simulink model "athree_phase_transestor_converter_hystersis"  (R2015a)
settings: Solver=ode45  StartTime=0.0  StopTime=0.1  RelTol=1e-3
libraries: simulink_extras x1
settings Model: Creator=Windows 10  LastModifiedBy=Windows 10

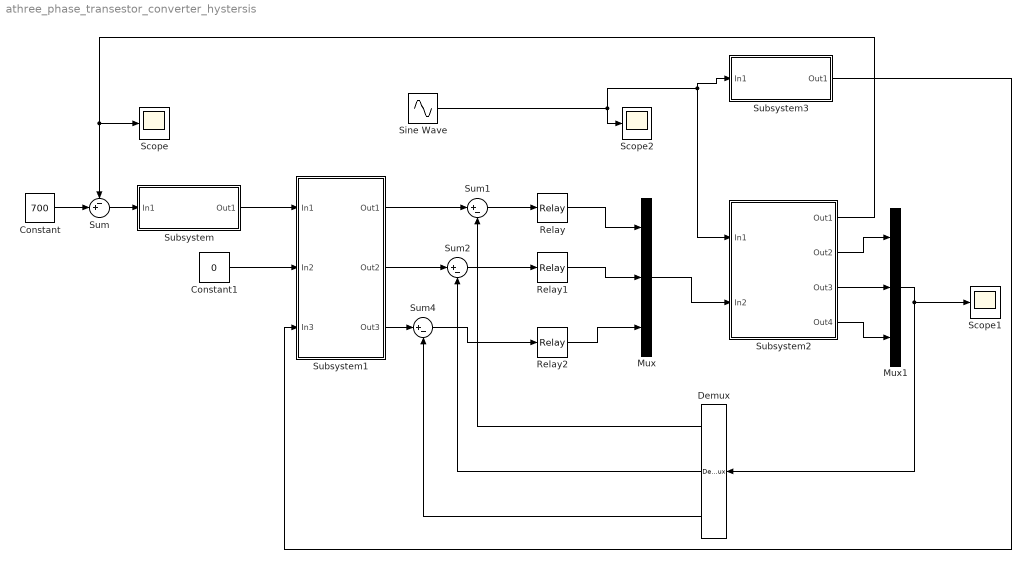
== system athree_phase_transestor_converter_hystersis ==
  Constant : Constant  Value=700
  Constant1 : Constant  Value=0
  Demux : Demux  Outputs=3
  Mux : Mux  Inputs=3
  Mux1 : Mux  Inputs=3
  Relay : Relay  OnSwitchValue=1  OffSwitchValue=-1  OnOutputValue=0  OffOutputValue=1
  Relay1 : Relay  OnSwitchValue=1  OffSwitchValue=-1  OnOutputValue=0  OffOutputValue=1
  Relay2 : Relay  OnSwitchValue=1  OffSwitchValue=-1  OnOutputValue=0  OffOutputValue=1
  Scope : Scope
  Scope1 : Scope
  Scope2 : Scope
      settings: SaveName=ScopeData2
  Sine Wave : Sin  Amplitude=326.5  Frequency=100*pi  Phase=[0 2*pi/3 4*pi/3]  SampleTime=0
  Subsystem : Subsystem
  Subsystem1 : Subsystem
  Subsystem2 : Subsystem
  Subsystem3 : Subsystem
  Sum : Sum  Inputs=-+|
  Sum1 : Sum  Inputs=|+-
  Sum2 : Sum  Inputs=|+-
  Sum4 : Sum  Inputs=|+-
  wires:
  Constant/1 -> Sum/2
  Sum/1 -> Subsystem/1(In1)
  Subsystem/1(Out1) -> Subsystem1/1(In1)
  Constant1/1 -> Subsystem1/2(In2)
  Subsystem1/1(Out1) -> Sum1/1
  Subsystem1/3(Out3) -> Sum4/1
  Subsystem1/2(Out2) -> Sum2/1
  Sum1/1 -> Relay/1
  Sum4/1 -> Relay2/1
  Sum2/1 -> Relay1/1
  Relay1/1 -> Mux/2
  Relay2/1 -> Mux/3
  Relay/1 -> Mux/1
  Demux/1 -> Sum1/2
  Demux/2 -> Sum2/2
  Demux/3 -> Sum4/2
  Subsystem3/1(Out1) -> Subsystem1/3(In3)
  Sine Wave/1 -> Subsystem3/1(In1), Subsystem2/1(In1), Scope2/1
  Mux/1 -> Subsystem2/2(In2)
  Subsystem2/2(Out2) -> Mux1/1
  Subsystem2/3(Out3) -> Mux1/2
  Subsystem2/4(Out4) -> Mux1/3
  Subsystem2/1(Out1) -> Sum/1, Scope/1
  Mux1/1 -> Scope1/1, Demux/1

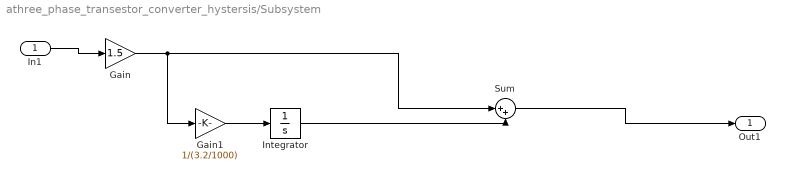
== system athree_phase_transestor_converter_hystersis/Subsystem ==
  In1 : Inport
  Gain : Gain  Gain=1.5
  Gain1 : Gain  Gain=1/(3.2/1000)
  Integrator : Integrator
  Sum : Sum  Inputs=|++
  Out1 : Outport
  wires:
  Gain1/1 -> Integrator/1
  Integrator/1 -> Sum/2
  Gain/1 -> Gain1/1, Sum/1
  In1/1 -> Gain/1
  Sum/1 -> Out1/1

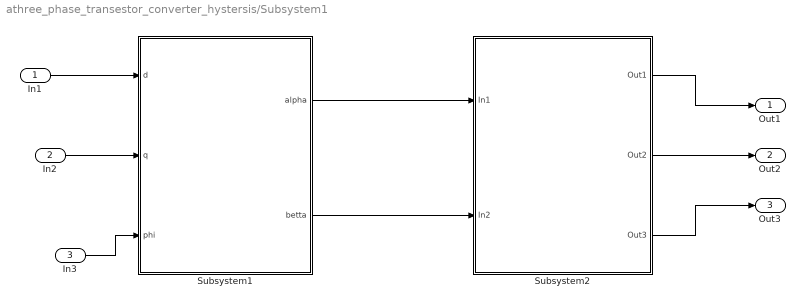
== system athree_phase_transestor_converter_hystersis/Subsystem1 ==
  In1 : Inport
  In2 : Inport  Port=2
  In3 : Inport  Port=3
  Subsystem1 : Subsystem
  Subsystem2 : Subsystem
  Out1 : Outport
  Out2 : Outport  Port=2
  Out3 : Outport  Port=3
  wires:
  Subsystem2/2(Out2) -> Out2/1
  Subsystem1/1(alpha) -> Subsystem2/1(In1)
  Subsystem2/3(Out3) -> Out3/1
  Subsystem2/1(Out1) -> Out1/1
  In3/1 -> Subsystem1/3(phi)
  In1/1 -> Subsystem1/1(d)
  In2/1 -> Subsystem1/2(q)
  Subsystem1/2(betta) -> Subsystem2/2(In2)

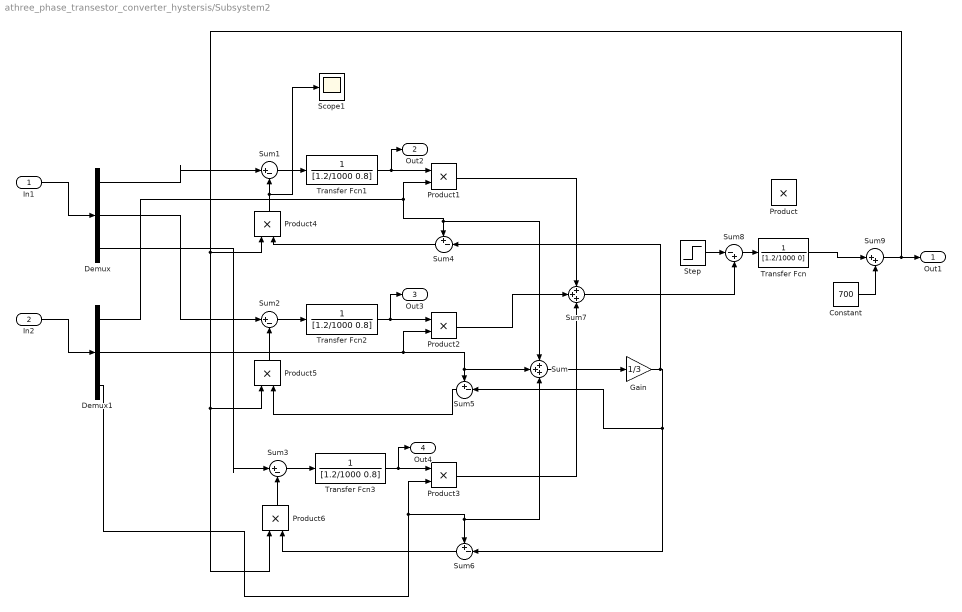
== system athree_phase_transestor_converter_hystersis/Subsystem2 ==
  In1 : Inport
  In2 : Inport  Port=2
  Constant : Constant  Value=700
  Demux : Demux  Outputs=3
  Demux1 : Demux  Outputs=3
  Gain : Gain  Gain=1/3
  Product{,1..6} (7 alike) : Product
  Scope1 : Scope
      settings: SaveName=ScopeData3
  Step : Step  Time=0.05  Before=15  After=30  SampleTime=0
  Sum : Sum  Inputs=+++
  Sum1 : Sum  Inputs=|+-
  Sum2 : Sum  Inputs=|+-
  Sum3 : Sum  Inputs=|+-
  Sum4 : Sum  Inputs=+-|
  Sum5 : Sum  Inputs=+-|
  Sum6 : Sum  Inputs=+-|
  Sum7 : Sum  Inputs=+++
  Sum8 : Sum  Inputs=|-+
  Sum9 : Sum  Inputs=|++
  Transfer Fcn : TransferFcn  Denominator=[1.2/1000 0]
  Transfer Fcn1 : TransferFcn  Denominator=[1.2/1000 0.8]
  Transfer Fcn2 : TransferFcn  Denominator=[1.2/1000 0.8]
  Transfer Fcn3 : TransferFcn  Denominator=[1.2/1000 0.8]
  Out1 : Outport
  Out2 : Outport  Port=2
  Out3 : Outport  Port=3
  Out4 : Outport  Port=4
  wires:
  In1/1 -> Demux/1
  In2/1 -> Demux1/1
  Sum1/1 -> Transfer Fcn1/1
  Sum2/1 -> Transfer Fcn2/1
  Sum3/1 -> Transfer Fcn3/1
  Demux/1 -> Sum1/1
  Demux/2 -> Sum2/1
  Demux/3 -> Sum3/1
  Transfer Fcn1/1 -> Out2/1, Product1/1
  Transfer Fcn2/1 -> Out3/1, Product2/1
  Transfer Fcn3/1 -> Out4/1, Product3/1
  Product4/1 -> Scope1/1, Sum1/2
  Product5/1 -> Sum2/2
  Product6/1 -> Sum3/2
  Demux1/1 -> Sum/1, Sum4/1, Product1/2
  Sum4/1 -> Product4/2
  Sum5/1 -> Product5/2
  Sum6/1 -> Product6/2
  Demux1/2 -> Sum/2, Sum5/1, Product2/2
  Demux1/3 -> Sum/3, Sum6/1, Product3/2
  Product2/1 -> Sum7/2
  Product1/1 -> Sum7/1
  Product3/1 -> Sum7/3
  Sum7/1 -> Sum8/2
  Step/1 -> Sum8/1
  Sum8/1 -> Transfer Fcn/1
  Transfer Fcn/1 -> Sum9/1
  Constant/1 -> Sum9/2
  Sum9/1 -> Product4/1, Product5/1, Product6/1, Out1/1
  Sum/1 -> Gain/1
  Gain/1 -> Sum4/2, Sum5/2, Sum6/2

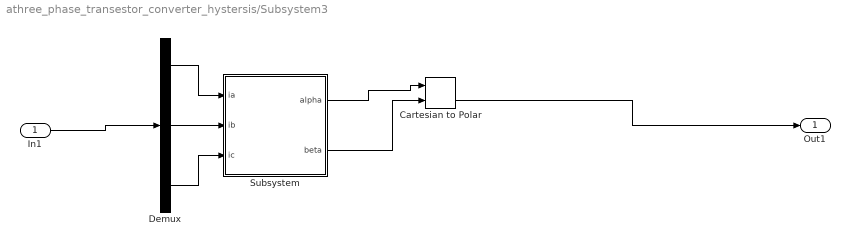
== system athree_phase_transestor_converter_hystersis/Subsystem3 ==
  In1 : Inport
  Cartesian to Polar : simulink_extras/Transformations/Cartesian to Polar
  Demux : Demux  Outputs=3
  Subsystem : Subsystem
  Out1 : Outport
  wires:
  Subsystem/1(alpha) -> Cartesian to Polar/1
  Subsystem/2(beta) -> Cartesian to Polar/2
  Cartesian to Polar/2 -> Out1/1
  In1/1 -> Demux/1
  Demux/1 -> Subsystem/1(ia)
  Demux/2 -> Subsystem/2(ib)
  Demux/3 -> Subsystem/3(ic)

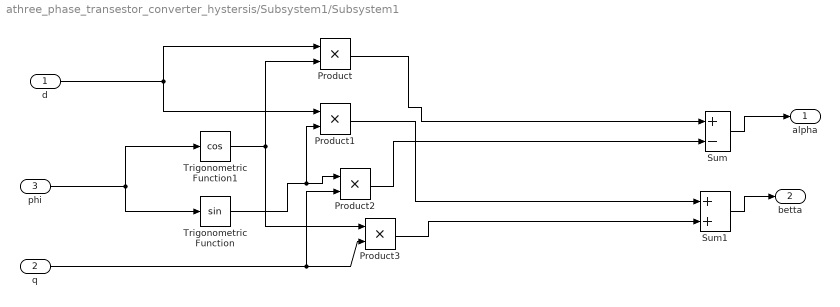
== system athree_phase_transestor_converter_hystersis/Subsystem1/Subsystem1 ==
  d : Inport
  q : Inport  Port=2
  phi : Inport  Port=3
  Product{,1..3} (4 alike) : Product
  Sum : Sum  Inputs=+-
  Sum1 : Sum
  Trigonometric Function : Trigonometry
  Trigonometric Function1 : Trigonometry  Operator=cos
  alpha : Outport
  betta : Outport  Port=2
  wires:
  Sum/1 -> alpha/1
  Sum1/1 -> betta/1
  phi/1 -> Trigonometric Function/1, Trigonometric Function1/1
  Product/1 -> Sum/1
  Product1/1 -> Sum1/1
  Product2/1 -> Sum/2
  Product3/1 -> Sum1/2
  q/1 -> Product2/2, Product3/2
  Trigonometric Function/1 -> Product1/2, Product2/1
  Trigonometric Function1/1 -> Product3/1, Product/2
  d/1 -> Product1/1, Product/1

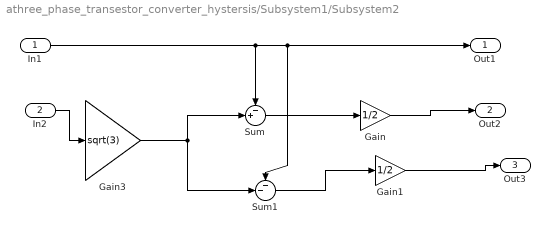
== system athree_phase_transestor_converter_hystersis/Subsystem1/Subsystem2 ==
  In1 : Inport
  In2 : Inport  Port=2
  Gain : Gain  Gain=1/2
  Gain1 : Gain  Gain=1/2
  Gain3 : Gain  Gain=sqrt(3)
  Sum : Sum  Inputs=-+|
  Sum1 : Sum  Inputs=--|
  Out1 : Outport
  Out2 : Outport  Port=2
  Out3 : Outport  Port=3
  wires:
  Gain/1 -> Out2/1
  Gain1/1 -> Out3/1
  In2/1 -> Gain3/1
  Gain3/1 -> Sum/2, Sum1/2
  In1/1 -> Sum1/1, Out1/1, Sum/1
  Sum/1 -> Gain/1
  Sum1/1 -> Gain1/1

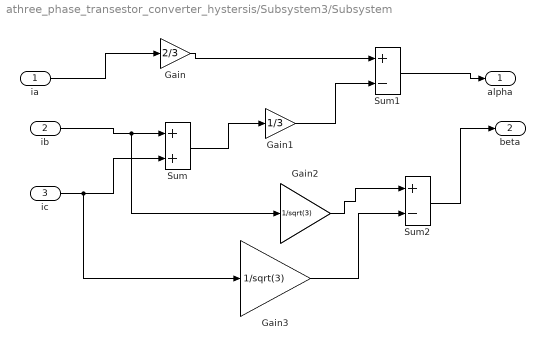
== system athree_phase_transestor_converter_hystersis/Subsystem3/Subsystem ==
  ia : Inport
  ib : Inport  Port=2
  ic : Inport  Port=3
  Gain : Gain  Gain=2/3
  Gain1 : Gain  Gain=1/3
  Gain2 : Gain  Gain=1/sqrt(3)
  Gain3 : Gain  Gain=1/sqrt(3)
  Sum : Sum
  Sum1 : Sum  Inputs=+-
  Sum2 : Sum  Inputs=+-
  alpha : Outport
  beta : Outport  Port=2
  wires:
  Sum1/1 -> alpha/1
  Sum2/1 -> beta/1
  Gain/1 -> Sum1/1
  Gain1/1 -> Sum1/2
  Sum/1 -> Gain1/1
  ia/1 -> Gain/1
  ib/1 -> Gain2/1, Sum/1
  ic/1 -> Gain3/1, Sum/2
  Gain2/1 -> Sum2/1
  Gain3/1 -> Sum2/2
